simulink model "sldemo_hydrod_org"  (Simulink 10.0)
settings: Solver=ode45  StartTime=0.0  StopTime=0.1  RelTol=1e-3  AbsTol=1e-6
model workspace (MATLAB code in the model file):
  | % Load the initial conditions and initialization data
  | % Using the same MAT file as
  | % sldemo_hydcyl
  | % sldemo_hydcyl4
  | % sldemo_hydrod
  | 
  | load sldemo_hydcyl_data;
undefined symbols (not defined in the file): Ac, C2, I, L, M, Qmax
libraries: hydlib x4, simulink x2
Description:
  | Two Cylinder Model with Load Constraints
  | 
  | In this model, a rigid rod supporting a large mass interconnects two
  | hydraulic actuators. The model eliminates the springs as it applies the
  | piston forces directly to the load. These forces balance the
  | gravitational force and result in both linear and rotational displacement.
  | See two related demos that use the same basic components:
  | 
  | * four cylinder model: sldemo_hydcyl4
  | * single cylinder model: sldemo_hydcyl
settings Model: Creator=The MathWorks, Inc.  LastModifiedBy=bhisma  ExtModeTrigMode=oneshot  ExtModeArmWhenConnect=off  ExtModeAutoUpdateStatusClock=off
settings SolverCC: AutoScaleAbsTol=off
settings DataIOCC: SaveFormat=Structure  SaveOutput=off  SaveState=on  SaveTime=off  ReturnWorkspaceOutputs=on  SignalLoggingName=sldemo_hydrod_output
settings OptimizationCC: BlockReduction=off  BooleanDataType=off  ExpressionDepthLimit=2147483647  InitFltsAndDblsToZero=on  BufferReusableBoundary=off
settings DebuggingCC: AlgebraicLoopMsg=none  SaveWithParameterizedLinksMsg=none  SignalResolutionControl=TryResolveAllWithWarning  MultiTaskDSMMsg=warning  MultiTaskCondExecSysMsg=none  SigSpecEnsureSampleTimeMsg=none  IntegerOverflowMsg=none  FcnCallInpInsideContextMsg=warning  BusObjectLabelMismatch=none  StateNameClashWarn=warning  IntegerSaturationMsg=none
settings HardwareCC: TargetUnknown=on
settings GRTTargetCC: TargetFcnLib=ansi_tfl_tmw.mat  GeneratePreprocessorConditionals=Disable all
settings ConfigComp: CovMetricSettings=d  CovExternalEMLEnable=off

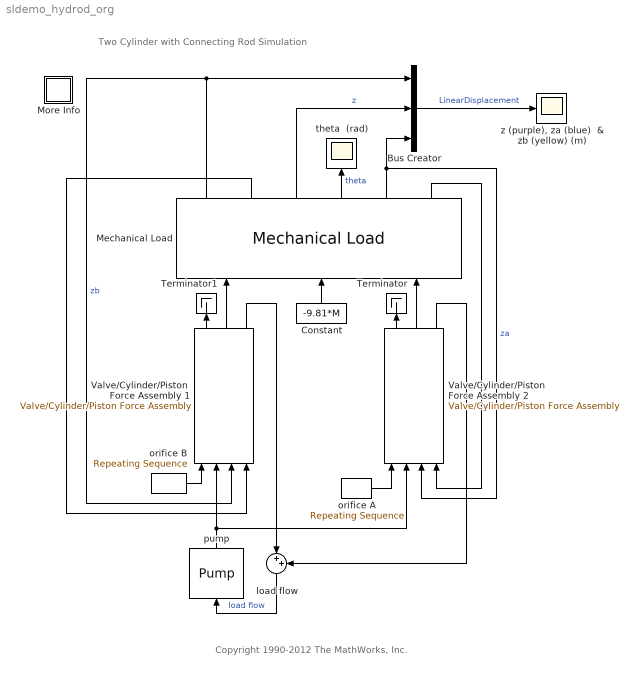
== system sldemo_hydrod_org ==
  note: Two Cylinder with Connecting Rod Simulation
  note: Copyright 1990-2012 The MathWorks, Inc.
  Bus Creator : BusCreator  Inputs=3
  Constant : Constant  Value=-9.81*M
  Mechanical Load : hydlib/Mechanical Load  L=L  M=M  I=I  zDotName=velocity  zName=displacement  thetaDotName=angular_velocity  thetaName=angular_displacement
  More Info : Subsystem
      settings: OpenFcn=showExample('simulink_general/sldemo_hydrodExample')
      mask Display: disp('?')
  Terminator : Terminator
  Terminator1 : Terminator
  Valve/Cylinder/Piston  Force Assembly 1 : hydlib/Valve//Cylinder//Piston Force Assembly  C1=C1  Ac=Ac  Cd=Cd  rho=rho  V30=V30  beta=Beta  p30=9.81*M/2/Ac  assemblyName=forceLeft
  Valve/Cylinder/Piston  Force Assembly 2 : hydlib/Valve//Cylinder//Piston Force Assembly  C1=C1  Ac=Ac  Cd=Cd  rho=rho  V30=V30  beta=Beta  p30=9.81*M/2/Ac  assemblyName=forceRight
  load flow : Sum  Inputs=|++  SaturateOnIntegerOverflow=on  InputSameDT=on  OutDataTypeStr=Inherit: Same as first input
  orifice A : simulink/Sources/Repeating Sequence  rep_seq_t="[0  0.1  0.2]/10"  rep_seq_y=[1 0 1]*1e-5
  orifice B : simulink/Sources/Repeating Sequence  rep_seq_t=[0 0.1 0.2]/10  rep_seq_y=[0 1 0]*1e-5
  pump : hydlib/Pump  t="[0        .04]"  Qpump=Qmax*[1 1]  p10=9.81*M/2/Ac  C2=C2/10
  theta  (rad) : Scope
  "z (purple), za (blue)  & zb (yellow) (m)" : Scope
  wires:
  Mechanical Load/1 -> Valve/Cylinder/Piston  Force Assembly 1/3, Bus Creator/1  "zb"
  Mechanical Load/5 -> Valve/Cylinder/Piston  Force Assembly 2/3, Bus Creator/3  "za"
  Mechanical Load/3 -> Bus Creator/2  "z"
  Mechanical Load/4 -> theta  (rad)/1  "theta"
  Constant/1 -> Mechanical Load/2
  Bus Creator/1 -> "z (purple), za (blue)  & zb (yellow) (m)"/1  "LinearDisplacement"
  Valve/Cylinder/Piston  Force Assembly 2/2 -> Mechanical Load/3
  Mechanical Load/6 -> Valve/Cylinder/Piston  Force Assembly 2/4
  orifice A/1 -> Valve/Cylinder/Piston  Force Assembly 2/1
  Valve/Cylinder/Piston  Force Assembly 2/1 -> Terminator/1
  Valve/Cylinder/Piston  Force Assembly 1/2 -> Mechanical Load/1
  Mechanical Load/2 -> Valve/Cylinder/Piston  Force Assembly 1/4
  orifice B/1 -> Valve/Cylinder/Piston  Force Assembly 1/1
  Valve/Cylinder/Piston  Force Assembly 1/1 -> Terminator1/1
  pump/1 -> Valve/Cylinder/Piston  Force Assembly 1/2, Valve/Cylinder/Piston  Force Assembly 2/2
  load flow/1 -> pump/1  "load flow"
  Valve/Cylinder/Piston  Force Assembly 2/3 -> load flow/2
  Valve/Cylinder/Piston  Force Assembly 1/3 -> load flow/1

== system sldemo_hydrod_org/More Info ==
